simulink model "Practice_simulink"  (R2015a)
settings: Solver=ode45  StartTime=0.0  StopTime=20  RelTol=1e-3
settings Model: Creator=DELL  LastModifiedBy=DELL

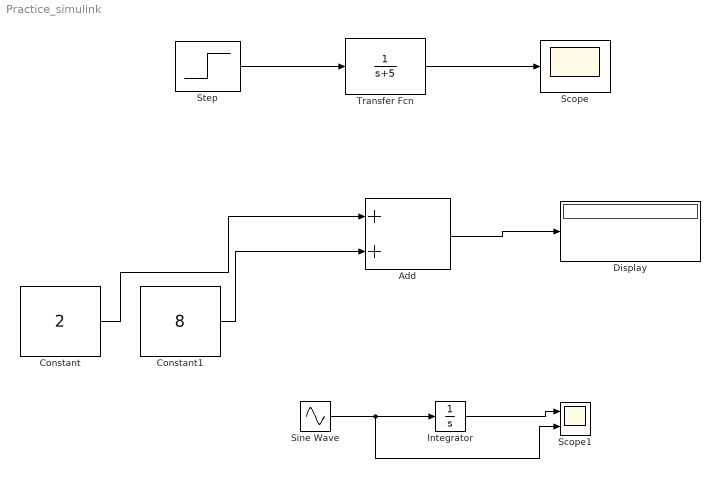
== system Practice_simulink ==
  Add : Sum
  Constant : Constant  Value=2
  Constant1 : Constant  Value=8
  Display : Display
  Integrator : Integrator
  Scope : Scope
      settings: TimeRange=5  YMin=0  YMax=0.2
  Scope1 : Scope  NumInputPorts=2
      settings: YMin=-5~-5  YMax=5~5
  Sine Wave : Sin  SampleTime=0
  Step : Step  SampleTime=0
  Transfer Fcn : TransferFcn  Denominator=[1 5]
  wires:
  Constant/1 -> Add/1
  Constant1/1 -> Add/2
  Add/1 -> Display/1
  Step/1 -> Transfer Fcn/1
  Transfer Fcn/1 -> Scope/1
  Sine Wave/1 -> Scope1/2, Integrator/1
  Integrator/1 -> Scope1/1
